simulink model "assi2_q1b_simu"  (R2022a)
settings: Solver=VariableStepAuto  StartTime=0.0  StopTime=10e4  RelTol=1e-3
undefined symbols (not defined in the file): m, n
settings Model: Creator=Yinhao  LastModifiedBy=Yinhao

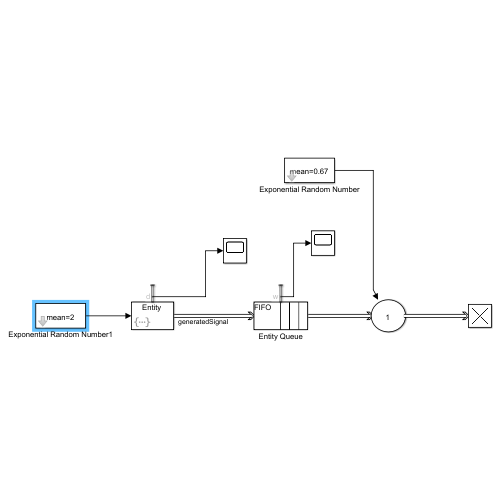
[thumbnail: Simulink's stored preview of the top-level diagram]
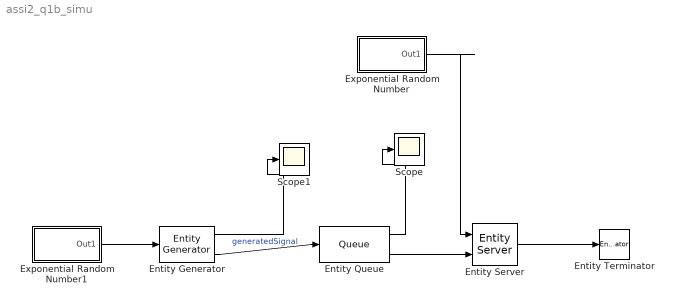
== system assi2_q1b_simu ==
  Entity Generator : EntityGenerator  OutputPortMessageModes=n,m  TimeSource=Signal port  GenerateAction=|  AttributeName=pass  NumberEntitiesDeparted=on  EntityType=Structured  EntityTypeName=Entity
      | persistent count;
      | if isempty(count)
      |     count = 0;
      | end
      | if(count>100)
      |     entity.pass = -1;
      | else
      |     count = count + 1;
      | end
      settings: InputPortMap=u1  OutputPortMap=o0,o3
  Entity Queue : Queue  InputPortMessageModes=m  OutputPortMessageModes=n,m  Capacity=1000  AverageWait=on
      settings: OutputPortMap=o2,o5
  Entity Server : EntityServer  InputPortMessageModes=n,m  OutputPortMessageModes=m  Capacity=1  ServiceTimeSource=Signal port  ServiceTimeValue=2/3
      settings: InputPortMap=u0,u2
  Entity Terminator : EntityTerminator  InputPortMessageModes=m
  Exponential Random Number : Subsystem  mask(Exponential Random Number){mean=0.67, seed=888}
      mask prompts: seed "Random Seed"
      mask help: This block generate a random number with exponential distribution.
      mask Display: disp(['mean=' num2str(mean,2)],"texmode","on");
  Exponential Random Number1 : Subsystem  mask(Exponential Random Number){mean=2, seed=777}
      mask prompts: seed "Random Seed"
      mask help: This block generate a random number with exponential distribution.
      mask Display: disp(['mean=' num2str(mean,2)],"texmode","on");
  Scope : Scope
  Scope1 : Scope
  wires:
  Entity Queue/2 -> Entity Server/2
  Entity Server/1 -> Entity Terminator/1
  Entity Queue/1 -> Scope/1
  Exponential Random Number/1(Out1) -> Entity Server/1
  Exponential Random Number1/1(Out1) -> Entity Generator/1
  Entity Generator/1 -> Scope1/1
  Entity Generator/2 -> Entity Queue/1  "generatedSignal"

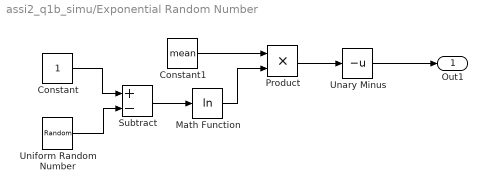
== system assi2_q1b_simu/Exponential Random Number ==
  Constant : Constant
  Constant1 : Constant  Value=mean
  Math Function : Math  Operator=log  SignedPower=on
  Product : Product  RndMeth=Zero
  Subtract : Sum  Inputs=+-
  Unary Minus : UnaryMinus
  Uniform Random Number : UniformRandomNumber  Minimum=0  Seed=seed
  Out1 : Outport
  wires:
  Subtract/1 -> Math Function/1
  Math Function/1 -> Product/2
  Unary Minus/1 -> Out1/1
  Product/1 -> Unary Minus/1
  Constant/1 -> Subtract/1
  Uniform Random Number/1 -> Subtract/2
  Constant1/1 -> Product/1

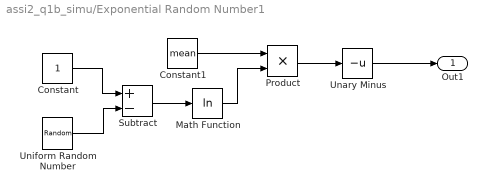
== system assi2_q1b_simu/Exponential Random Number1 ==
  Constant : Constant
  Constant1 : Constant  Value=mean
  Math Function : Math  Operator=log  SignedPower=on
  Product : Product  RndMeth=Zero
  Subtract : Sum  Inputs=+-
  Unary Minus : UnaryMinus
  Uniform Random Number : UniformRandomNumber  Minimum=0  Seed=seed
  Out1 : Outport
  wires:
  Subtract/1 -> Math Function/1
  Math Function/1 -> Product/2
  Unary Minus/1 -> Out1/1
  Product/1 -> Unary Minus/1
  Constant/1 -> Subtract/1
  Uniform Random Number/1 -> Subtract/2
  Constant1/1 -> Product/1
